simulink model "SAS_pitch_damper"  (R2020a)
settings: Solver=VariableStepAuto  StartTime=0.0  StopTime=10  RelTol=1e-3
settings Model: Creator=parth  LastModifiedBy=parth

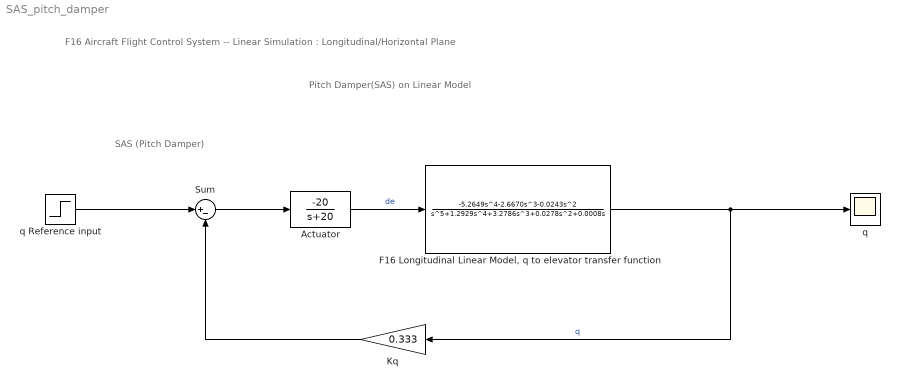
== system SAS_pitch_damper ==
  note: SAS (Pitch Damper)
  note: Pitch Damper(SAS) on Linear Model
  note: F16 Aircraft Flight Control System -- Linear Simulation : Longitudinal/Horizontal Plane
  Actuator : TransferFcn  Numerator=[-20]  Denominator=[1, 20]
  "F16 Longitudinal Linear Model, q to elevator transfer function" : TransferFcn  Numerator="[0   -5.2649   -2.6670   -0.0243   -0.0000 0.000]"  Denominator="[1.0000    1.2929    3.2786    0.0278    0.0008 0.000]"
  Kq : Gain  Gain=0.333
  Sum : Sum  Inputs=|+-
  q : Scope
  q Reference input : Step  Time=0  SampleTime=0
  wires:
  Actuator/1 -> "F16 Longitudinal Linear Model, q to elevator transfer function"/1  "de"
  "F16 Longitudinal Linear Model, q to elevator transfer function"/1 -> q/1, Kq/1  "q"
  q Reference input/1 -> Sum/1
  Kq/1 -> Sum/2
  Sum/1 -> Actuator/1
